simulink model "active_suspension_block_diagram"  (R2024b)
settings: Solver=ode45  StartTime=0.0  StopTime=60  RelTol=1e-3  AbsTol=1e-6
values from neighbouring files (symbols this model uses):
  a = 0.078    [param.m]
  bs = 0    [param.m]
  bus = 0    [param.m]
  F = 0.3    [param.m]
  K = lqr( A, B(:,2), Q, R )    [param.m]
  ks = 6921    [param.m]
  kus = 81000    [param.m]
  ms = 34    [param.m]
  mus = 11    [param.m]
settings Model: Creator=Rick  LastModifiedBy=rob
settings SolverCC: AutoScaleAbsTol=off  AlgebraicLoopSolver=TrustRegion
settings DataIOCC: SaveFormat=Array  SignalLoggingSaveFormat=ModelDataLogs  ReturnWorkspaceOutputs=off
settings OptimizationCC: BlockReduction=off  BooleanDataType=off  ExpressionDepthLimit=2147483647  LifeSpan=inf
settings DebuggingCC: SaveWithParameterizedLinksMsg=none  UnderspecifiedInitializationDetection=Classic  MergeDetectMultiDrivingBlocksExec=none  SignalResolutionControl=TryResolveAllWithWarning  InheritedTsInSrcMsg=none  MultiTaskDSMMsg=warning  MultiTaskCondExecSysMsg=none  FcnCallInpInsideContextMsg=warning  UnconnectedInputMsg=warning  UnconnectedOutputMsg=warning  UnconnectedLineMsg=warning  UnknownTsInhSupMsg=none  StateNameClashWarn=warning  SFUnexpectedBacktrackingDiag=warning  SFNoUnconditionalDefaultTransitionDiag=warning  SFExecutionAtInitializationDiag=none  ArithmeticOperatorsInVariantConditions=warning
settings HardwareCC: ProdBitPerPointer=32  ProdBitPerSizeT=32  ProdBitPerPtrDiffT=32  ProdLargestAtomicFloat=None  ProdIntDivRoundTo=Undefined  ProdEndianess=Unspecified  ProdWordSize=32  ProdHWDeviceType=32-bit Generic  TargetUnknown=on
settings ModelReferenceCC: PropagateSignalLabelsOutOfModel=off
settings SFSimCC: SimUseLocalCustomCode=off  CustomCodeUndefinedFunction=UseInterfaceOnly
settings RTWCC: RTWUseLocalCustomCode=off  GPUComputeCapability=3.5
settings CodeAppCC: StateflowObjectComments=on
settings GRTTargetCC: TargetLangStandard=C89/C90 (ANSI)
settings ConfigComp: CovMetricSettings=dw  CovSaveCumulativeToWorkspaceVar=on  CovSaveSingleToWorkspaceVar=on  CovExternalEMLEnable=off

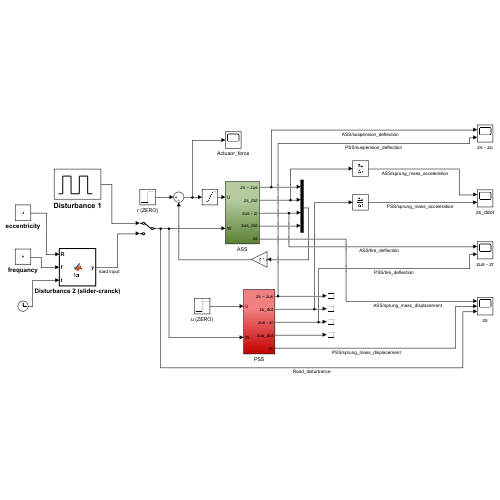
[thumbnail: Simulink's stored preview of the top-level diagram]
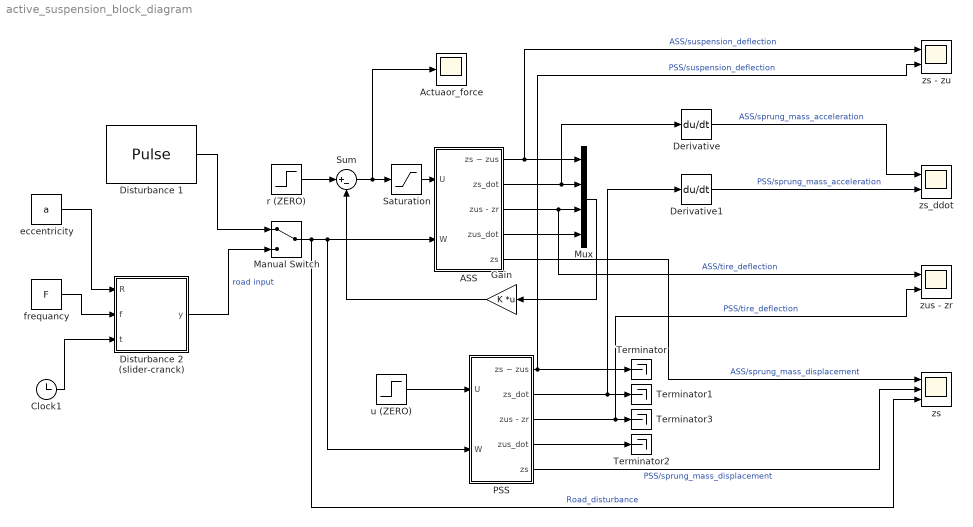
== system active_suspension_block_diagram ==
  ASS : Subsystem
  Actuaor_force : Scope
  Clock1 : Clock
      settings: Decimation=Sim_Time
  Derivative : Derivative
  Derivative1 : Derivative
  Disturbance 1 : DiscretePulseGenerator  PulseType=Time based  Amplitude=0.1  Period=6  PulseWidth=50  PhaseDelay=.1
  Disturbance 2 (slider-cranck) : MATLAB Function  TreatAsAtomicUnit=on
  Gain : Gain  Gain=K  Multiplication=Matrix(K*u)
  Manual Switch : ManualSwitch
  Mux : Mux
  PSS : Subsystem
  Saturation : Saturate  UpperLimit=250  LowerLimit=-250
  Sum : Sum  Inputs=|+-
  Terminator{,1..3} (4 alike) : Terminator
  eccentricity : Constant  Value=a
  frequancy : Constant  Value=F
  r (ZERO) : Step  Time=0  After=0  SampleTime=0
  u (ZERO) : Step  Time=0  After=0  SampleTime=0
  zs : Scope  NumInputPorts=3
  zs - zu : Scope  NumInputPorts=2
  zs_ddot : Scope  NumInputPorts=2
  zus - zr : Scope  NumInputPorts=2
  wires:
  ASS/2(zs_dot) -> Derivative/1, Mux/2
  ASS/4(zus_dot) -> Mux/4
  Mux/1 -> Gain/1
  Gain/1 -> Sum/2
  eccentricity/1 -> Disturbance 2 (slider-cranck)/1(R)
  frequancy/1 -> Disturbance 2 (slider-cranck)/2(f)
  Clock1/1 -> Disturbance 2 (slider-cranck)/3(t)
  Disturbance 2 (slider-cranck)/1(y) -> Manual Switch/2  "road input"
  r (ZERO)/1 -> Sum/1
  Disturbance 1/1 -> Manual Switch/1
  u (ZERO)/1 -> PSS/1(U)
  Manual Switch/1 -> zs/3, PSS/2(W), ASS/2(W)  "Road_disturbance"
  PSS/4(zus_dot) -> Terminator2/1
  PSS/2(zs_dot) -> Derivative1/1, Terminator1/1
  PSS/3(zus - zr) -> zus - zr/2, Terminator3/1  "PSS/tire_deflection"
  Sum/1 -> Saturation/1, Actuaor_force/1
  ASS/1(zs − zus) -> Mux/1, zs - zu/1  "ASS/suspension_deflection"
  PSS/1(zs − zus) -> Terminator/1, zs - zu/2  "PSS/suspension_deflection"
  ASS/3(zus - zr) -> zus - zr/1, Mux/3  "ASS/tire_deflection"
  Derivative1/1 -> zs_ddot/2  "PSS/sprung_mass_acceleration"
  Derivative/1 -> zs_ddot/1  "ASS/sprung_mass_acceleration"
  ASS/5(zs) -> zs/1  "ASS/sprung_mass_displacement"
  PSS/5(zs) -> zs/2  "PSS/sprung_mass_displacement"
  Saturation/1 -> ASS/1(U)

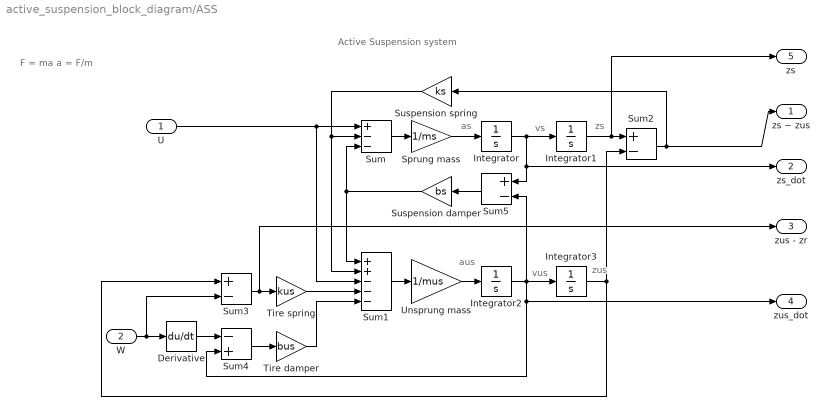
== system active_suspension_block_diagram/ASS ==
  note: Active Suspension system
  note: F = ma
      | a = F/m
  note: as
  note: vs
  note: zs
  note: aus
  note: vus
  note: zus
  U : Inport
  W : Inport  Port=2
  Derivative : Derivative
  Integrator{,1..3} (4 alike) : Integrator
  Sprung mass : Gain  Gain=1/ms  SaturateOnIntegerOverflow=on  OutDataTypeStr=Inherit: Same as input  ParamDataTypeStr=Inherit: Same as input
  Sum : Sum  Inputs=+--  InputSameDT=on  SaturateOnIntegerOverflow=on  OutDataTypeStr=Inherit: Same as first input
  Sum1 : Sum  Inputs=++---  InputSameDT=on  SaturateOnIntegerOverflow=on  OutDataTypeStr=Inherit: Same as first input
  Sum2 : Sum  Inputs=+-  InputSameDT=on  SaturateOnIntegerOverflow=on  OutDataTypeStr=Inherit: Same as first input
  Sum3 : Sum  Inputs=+-  InputSameDT=on  SaturateOnIntegerOverflow=on  OutDataTypeStr=Inherit: Same as first input
  Sum4 : Sum  Inputs=-+  InputSameDT=on  SaturateOnIntegerOverflow=on  OutDataTypeStr=Inherit: Same as first input
  Sum5 : Sum  Inputs=+-  InputSameDT=on  SaturateOnIntegerOverflow=on  OutDataTypeStr=Inherit: Same as first input
  Suspension damper : Gain  Gain=bs  SaturateOnIntegerOverflow=on  OutDataTypeStr=Inherit: Same as input  ParamDataTypeStr=Inherit: Same as input
  Suspension spring : Gain  Gain=ks  SaturateOnIntegerOverflow=on  OutDataTypeStr=Inherit: Same as input  ParamDataTypeStr=Inherit: Same as input
  Tire damper : Gain  Gain=bus  SaturateOnIntegerOverflow=on  OutDataTypeStr=Inherit: Same as input  ParamDataTypeStr=Inherit: Same as input
  Tire spring : Gain  Gain=kus  SaturateOnIntegerOverflow=on  OutDataTypeStr=Inherit: Same as input  ParamDataTypeStr=Inherit: Same as input
  Unsprung mass : Gain  Gain=1/mus  SaturateOnIntegerOverflow=on  OutDataTypeStr=Inherit: Same as input  ParamDataTypeStr=Inherit: Same as input
  zs − zus : Outport
  zs_dot : Outport  Port=2
  zus - zr : Outport  Port=3
  zus_dot : Outport  Port=4
  zs : Outport  Port=5
  wires:
  Suspension spring/1 -> Sum/2, Sum1/2
  Sprung mass/1 -> Integrator/1
  Sum2/1 -> zs − zus/1, Suspension spring/1
  Integrator/1 -> Sum5/1, zs_dot/1, Integrator1/1
  W/1 -> Sum3/2, Derivative/1
  Unsprung mass/1 -> Integrator2/1
  Derivative/1 -> Sum4/1
  Sum1/1 -> Unsprung mass/1
  Integrator1/1 -> zs/1, Sum2/1
  Suspension damper/1 -> Sum1/1, Sum/3
  Tire damper/1 -> Sum1/5
  Integrator2/1 -> Integrator3/1, Sum4/2, zus_dot/1, Sum5/2
  U/1 -> Sum1/3, Sum/1
  Sum3/1 -> zus - zr/1, Tire spring/1
  Sum5/1 -> Suspension damper/1
  Sum4/1 -> Tire damper/1
  Tire spring/1 -> Sum1/4
  Sum/1 -> Sprung mass/1
  Integrator3/1 -> Sum2/2, Sum3/1

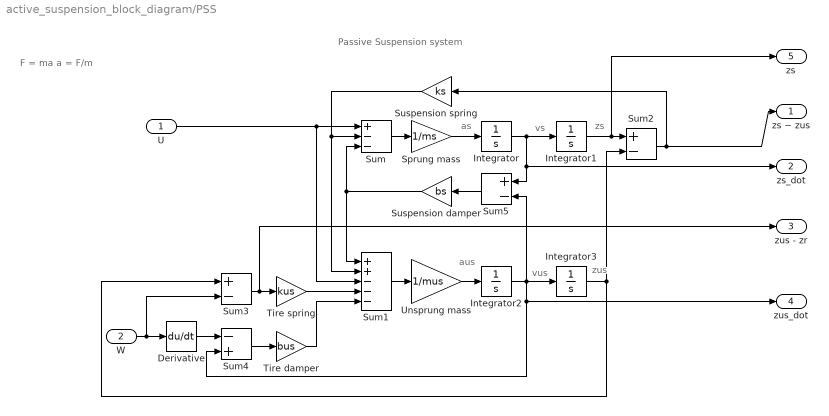
== system active_suspension_block_diagram/PSS ==
  note: zus
  note: vs
  note: zs
  note: as
  note: F = ma
      | a = F/m
  note: aus
  note: vus
  note: Passive Suspension system
  U : Inport
  W : Inport  Port=2
  Derivative : Derivative
  Integrator{,1..3} (4 alike) : Integrator
  Sprung mass : Gain  Gain=1/ms  SaturateOnIntegerOverflow=on  OutDataTypeStr=Inherit: Same as input  ParamDataTypeStr=Inherit: Same as input
  Sum : Sum  Inputs=+--  InputSameDT=on  SaturateOnIntegerOverflow=on  OutDataTypeStr=Inherit: Same as first input
  Sum1 : Sum  Inputs=++---  InputSameDT=on  SaturateOnIntegerOverflow=on  OutDataTypeStr=Inherit: Same as first input
  Sum2 : Sum  Inputs=+-  InputSameDT=on  SaturateOnIntegerOverflow=on  OutDataTypeStr=Inherit: Same as first input
  Sum3 : Sum  Inputs=+-  InputSameDT=on  SaturateOnIntegerOverflow=on  OutDataTypeStr=Inherit: Same as first input
  Sum4 : Sum  Inputs=-+  InputSameDT=on  SaturateOnIntegerOverflow=on  OutDataTypeStr=Inherit: Same as first input
  Sum5 : Sum  Inputs=+-  InputSameDT=on  SaturateOnIntegerOverflow=on  OutDataTypeStr=Inherit: Same as first input
  Suspension damper : Gain  Gain=bs  SaturateOnIntegerOverflow=on  OutDataTypeStr=Inherit: Same as input  ParamDataTypeStr=Inherit: Same as input
  Suspension spring : Gain  Gain=ks  SaturateOnIntegerOverflow=on  OutDataTypeStr=Inherit: Same as input  ParamDataTypeStr=Inherit: Same as input
  Tire damper : Gain  Gain=bus  SaturateOnIntegerOverflow=on  OutDataTypeStr=Inherit: Same as input  ParamDataTypeStr=Inherit: Same as input
  Tire spring : Gain  Gain=kus  SaturateOnIntegerOverflow=on  OutDataTypeStr=Inherit: Same as input  ParamDataTypeStr=Inherit: Same as input
  Unsprung mass : Gain  Gain=1/mus  SaturateOnIntegerOverflow=on  OutDataTypeStr=Inherit: Same as input  ParamDataTypeStr=Inherit: Same as input
  zs − zus : Outport
  zs_dot : Outport  Port=2
  zus - zr : Outport  Port=3
  zus_dot : Outport  Port=4
  zs : Outport  Port=5
  wires:
  Derivative/1 -> Sum4/1
  Sum/1 -> Sprung mass/1
  W/1 -> Sum3/2, Derivative/1
  Integrator3/1 -> Sum2/2, Sum3/1
  U/1 -> Sum1/3, Sum/1
  Integrator2/1 -> Integrator3/1, Sum4/2, zus_dot/1, Sum5/2
  Integrator/1 -> Sum5/1, zs_dot/1, Integrator1/1
  Unsprung mass/1 -> Integrator2/1
  Integrator1/1 -> zs/1, Sum2/1
  Suspension damper/1 -> Sum1/1, Sum/3
  Sum1/1 -> Unsprung mass/1
  Sum3/1 -> zus - zr/1, Tire spring/1
  Tire spring/1 -> Sum1/4
  Sum4/1 -> Tire damper/1
  Tire damper/1 -> Sum1/5
  Sum5/1 -> Suspension damper/1
  Suspension spring/1 -> Sum/2, Sum1/2
  Sprung mass/1 -> Integrator/1
  Sum2/1 -> zs − zus/1, Suspension spring/1

== matlab function active_suspension_block_diagram/Disturbance 2 (slider-cranck) ==
  data: y output; R input; f input; t input
function y = fcn(R,f,t)
% R eccentricity
% f frequancy 
% t time
omega = 2 * pi*f;
L=0.43; %length of connecting road
n=L/R;
theta = (omega * t*180)/pi;
x = R* ((1-cosd(theta+90)) + (n-sqrt(n^2 - sind(theta+90).^2)))-R*((1-cosd(90)) + (n-sqrt(n^2 - sind(90).^2)));y = x;
